simulink subsystem "Component4"  (R2022a)
settings: Solver=VariableStepAuto  StartTime=0.0  StopTime=10.0  RelTol=1e-3
settings Model: Creator=jdelolmo  LastModifiedBy=jdelolmo

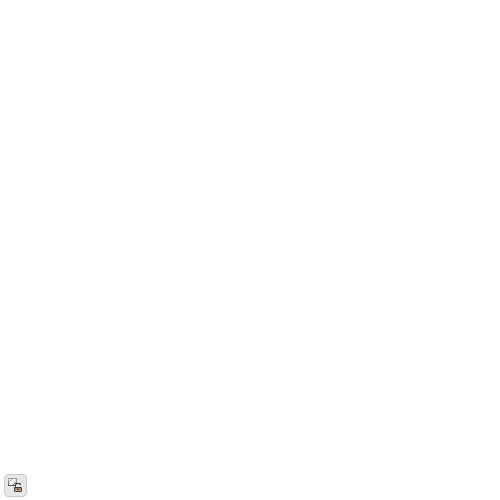
[thumbnail: Simulink's stored preview of the top-level diagram]
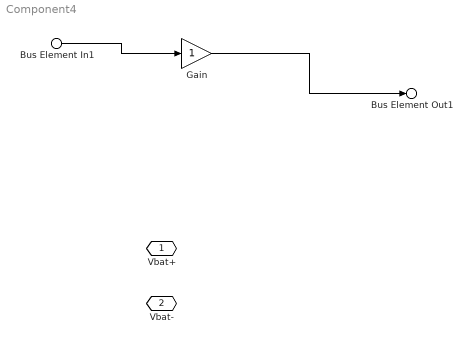
== system Component4 ==
  Bus Element In1 : Inport  PortName=InBus  Element=signal1
  Gain : Gain
  Vbat+ : PMIOPort  Side=Left
  Vbat- : PMIOPort  Port=2  Side=Left
  Bus Element Out1 : Outport  PortName=OutBus  Element=signal1
  wires:
  Bus Element In1/1 -> Gain/1
  Gain/1 -> Bus Element Out1/1
